simulink model "NonLinear_Plant"  (R2018a)
settings: Solver=VariableStepAuto  StartTime=0.0  StopTime=10.0  RelTol=1e-3
values from neighbouring files (symbols this model uses):
  Beta = 2.29e-06    [Plantvw.m]
  d = d    [Plantvw.m]
  dw = dw    [Plantsdv.m]    (also in Plantvw.m; Plantww.m)
  Kb = Kt    (= 0.0046)    [Plantvw.m]
  Kg = 50    [Plantvw.m]
  Kt = 0.0046    [Plantvw.m]
  La = 1.729e-03    (= 0.001729)    [Plantvw.m]
  mc = 2.76 + md    [Plantvw.m]
  R = R    [Plantww.m]
  Ra = 5.51    [Plantvw.m]
undefined symbols (not defined in the file or in its folder): Ad, Bd
settings Model: Creator=shravan  LastModifiedBy=shravan

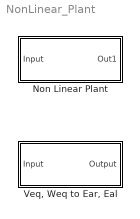
== system NonLinear_Plant ==
  "Non Linear Plant " : Subsystem
  "Veq, Weq to Ear, Eal " : Subsystem

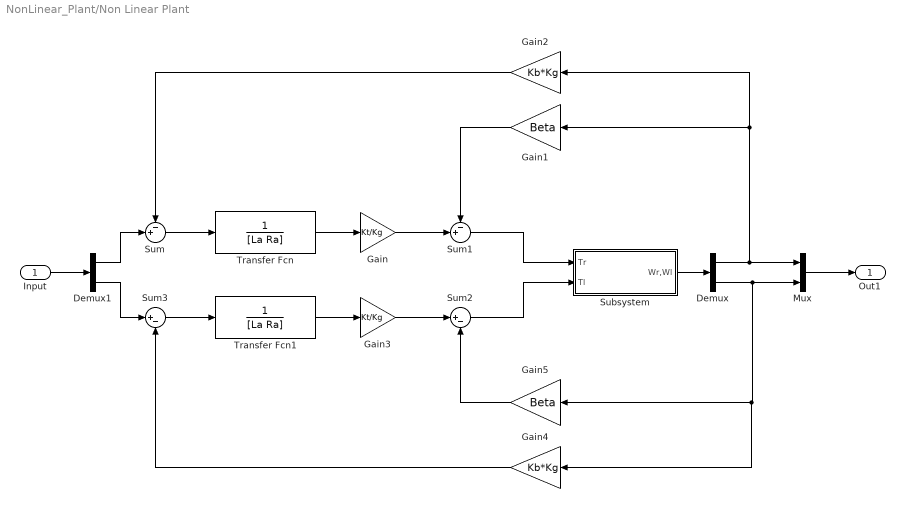
== system NonLinear_Plant/Non Linear Plant  ==
  Input : Inport
  Demux : Demux  Outputs=2
  Demux1 : Demux  Outputs=2
  Gain : Gain  Gain=Kt/Kg
  Gain1 : Gain  Gain=Beta
  Gain2 : Gain  Gain=Kb*Kg
  Gain3 : Gain  Gain=Kt/Kg
  Gain4 : Gain  Gain=Kb*Kg
  Gain5 : Gain  Gain=Beta
  Mux : Mux  Inputs=2
  Subsystem : Subsystem
  Sum : Sum  Inputs=-+|
  Sum1 : Sum  Inputs=-+|
  Sum2 : Sum  Inputs=|+-
  Sum3 : Sum  Inputs=|+-
  Transfer Fcn : TransferFcn  Denominator=[La Ra]
  Transfer Fcn1 : TransferFcn  Denominator=[La Ra]
  Out1 : Outport
  wires:
  Gain5/1 -> Sum2/2
  Gain4/1 -> Sum3/2
  Sum/1 -> Transfer Fcn/1
  Demux1/2 -> Sum3/1
  Gain1/1 -> Sum1/1
  Demux/1 -> Mux/1, Gain2/1, Gain1/1
  Subsystem/1(Wr,Wl) -> Demux/1
  Demux1/1 -> Sum/2
  Sum3/1 -> Transfer Fcn1/1
  Mux/1 -> Out1/1
  Gain2/1 -> Sum/1
  Gain/1 -> Sum1/2
  Input/1 -> Demux1/1
  Sum1/1 -> Subsystem/1(Tr)
  Transfer Fcn/1 -> Gain/1
  Transfer Fcn1/1 -> Gain3/1
  Gain3/1 -> Sum2/1
  Demux/2 -> Mux/2, Gain4/1, Gain5/1
  Sum2/1 -> Subsystem/2(Tl)

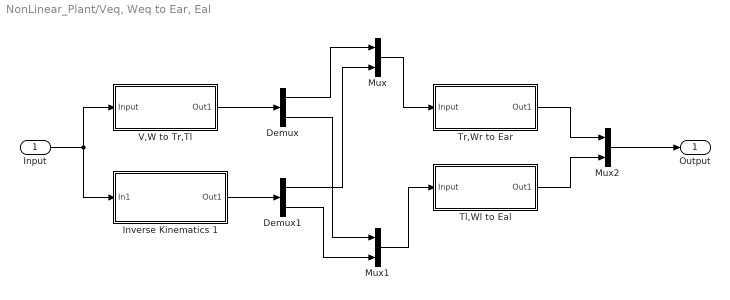
== system NonLinear_Plant/Veq, Weq to Ear, Eal  ==
  Input : Inport
  Demux : Demux  Outputs=2
  Demux1 : Demux  Outputs=2
  Inverse Kinematics 1 : Subsystem
  Mux : Mux  Inputs=2
  Mux1 : Mux  Inputs=2
  Mux2 : Mux  Inputs=2
  Tl,Wl to Eal : Subsystem
  Tr,Wr to Ear : Subsystem
  V,W to Tr,Tl : Subsystem
  Output : Outport
  wires:
  V,W to Tr,Tl/1(Out1) -> Demux/1
  Demux/1 -> Mux/1
  Mux/1 -> Tr,Wr to Ear/1(Input)
  Input/1 -> Inverse Kinematics 1/1(In1), V,W to Tr,Tl/1(Input)
  Inverse Kinematics 1/1(Out1) -> Demux1/1
  Demux1/1 -> Mux/2
  Demux/2 -> Mux1/1
  Demux1/2 -> Mux1/2
  Mux1/1 -> Tl,Wl to Eal/1(Input)
  Tr,Wr to Ear/1(Out1) -> Mux2/1
  Tl,Wl to Eal/1(Out1) -> Mux2/2
  Mux2/1 -> Output/1

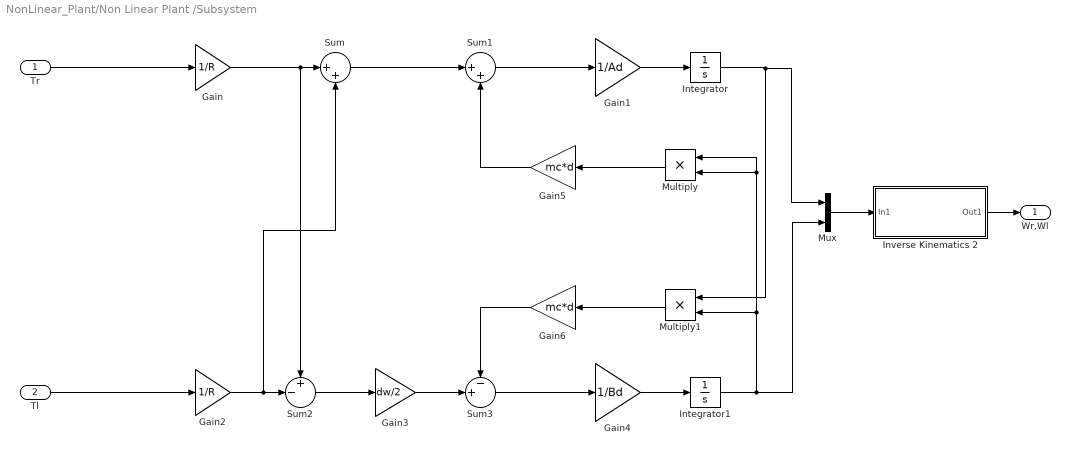
== system NonLinear_Plant/Non Linear Plant /Subsystem ==
  Tr : Inport
  Tl : Inport  Port=2
  Gain : Gain  Gain=1/R
  Gain1 : Gain  Gain=1/Ad
  Gain2 : Gain  Gain=1/R
  Gain3 : Gain  Gain=dw/2
  Gain4 : Gain  Gain=1/Bd
  Gain5 : Gain  Gain=mc*d
  Gain6 : Gain  Gain=mc*d
  Integrator : Integrator
  Integrator1 : Integrator
  Inverse Kinematics 2 : Subsystem
  Multiply : Product
  Multiply1 : Product
  Mux : Mux  Inputs=2
  Sum : Sum  Inputs=|++
  Sum1 : Sum  Inputs=|++
  Sum2 : Sum  Inputs=+-|
  Sum3 : Sum  Inputs=-+|
  Wr,Wl : Outport
  wires:
  Sum1/1 -> Gain1/1
  Multiply1/1 -> Gain6/1
  Sum3/1 -> Gain4/1
  Gain/1 -> Sum/1, Sum2/1
  Integrator/1 -> Mux/1, Multiply1/1
  Mux/1 -> Inverse Kinematics 2/1(In1)
  Gain4/1 -> Integrator1/1
  Inverse Kinematics 2/1(Out1) -> Wr,Wl/1
  Sum/1 -> Sum1/1
  Gain5/1 -> Sum1/2
  Tr/1 -> Gain/1
  Integrator1/1 -> Multiply1/2, Multiply/2, Multiply/1, Mux/2
  Multiply/1 -> Gain5/1
  Gain3/1 -> Sum3/2
  Sum2/1 -> Gain3/1
  Gain2/1 -> Sum/2, Sum2/2
  Gain6/1 -> Sum3/1
  Tl/1 -> Gain2/1
  Gain1/1 -> Integrator/1

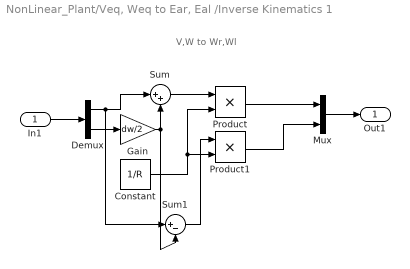
== system NonLinear_Plant/Veq, Weq to Ear, Eal /Inverse Kinematics 1 ==
  note: V,W to Wr,Wl
  In1 : Inport
  Constant : Constant  Value=1/R
  Demux : Demux  Outputs=2
  Gain : Gain  Gain=dw/2
  Mux : Mux  Inputs=2
  Product : Product
  Product1 : Product
  Sum : Sum  Inputs=|++
  Sum1 : Sum  Inputs=|+-
  Out1 : Outport
  wires:
  Mux/1 -> Out1/1
  In1/1 -> Demux/1
  Demux/2 -> Gain/1
  Demux/1 -> Sum1/1, Sum/1
  Sum/1 -> Product/1
  Constant/1 -> Product1/2, Product/2
  Sum1/1 -> Product1/1
  Product/1 -> Mux/1
  Product1/1 -> Mux/2
  Gain/1 -> Sum1/2, Sum/2

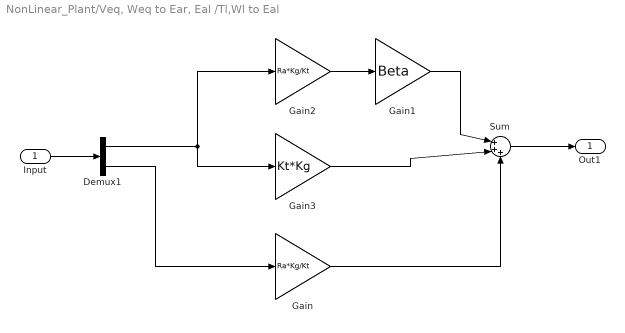
== system NonLinear_Plant/Veq, Weq to Ear, Eal /Tl,Wl to Eal ==
  Input : Inport
  Demux1 : Demux  Outputs=2
  Gain : Gain  Gain=Ra*Kg/Kt
  Gain1 : Gain  Gain=Beta
  Gain2 : Gain  Gain=Ra*Kg/Kt
  Gain3 : Gain  Gain=Kt*Kg
  Sum : Sum  Inputs=|+++
  Out1 : Outport
  wires:
  Demux1/1 -> Gain2/1, Gain3/1
  Gain/1 -> Sum/3
  Gain1/1 -> Sum/1
  Gain2/1 -> Gain1/1
  Input/1 -> Demux1/1
  Sum/1 -> Out1/1
  Demux1/2 -> Gain/1
  Gain3/1 -> Sum/2

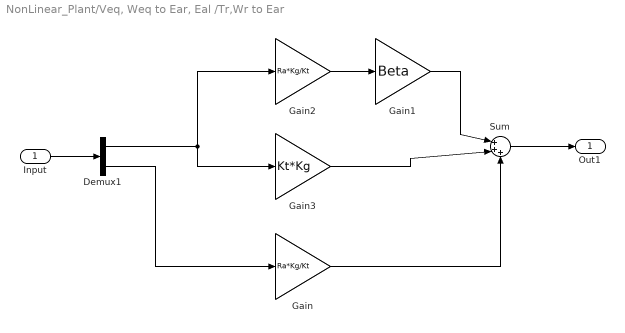
== system NonLinear_Plant/Veq, Weq to Ear, Eal /Tr,Wr to Ear ==
  Input : Inport
  Demux1 : Demux  Outputs=2
  Gain : Gain  Gain=Ra*Kg/Kt
  Gain1 : Gain  Gain=Beta
  Gain2 : Gain  Gain=Ra*Kg/Kt
  Gain3 : Gain  Gain=Kt*Kg
  Sum : Sum  Inputs=|+++
  Out1 : Outport
  wires:
  Demux1/1 -> Gain2/1, Gain3/1
  Gain/1 -> Sum/3
  Gain1/1 -> Sum/1
  Gain2/1 -> Gain1/1
  Input/1 -> Demux1/1
  Sum/1 -> Out1/1
  Demux1/2 -> Gain/1
  Gain3/1 -> Sum/2

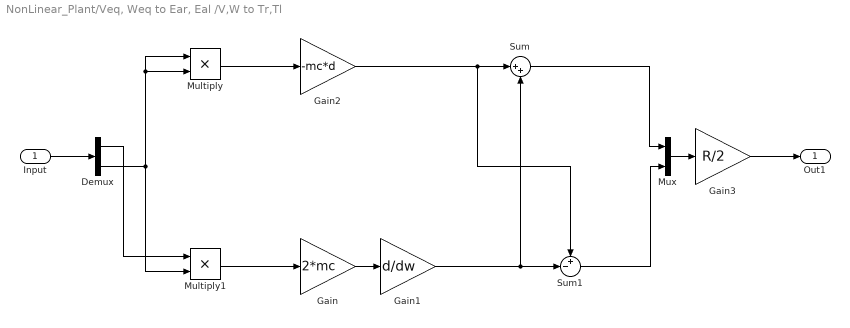
== system NonLinear_Plant/Veq, Weq to Ear, Eal /V,W to Tr,Tl ==
  Input : Inport
  Demux : Demux  Outputs=2
  Gain : Gain  Gain=2*mc
  Gain1 : Gain  Gain=d/dw
  Gain2 : Gain  Gain=-mc*d
  Gain3 : Gain  Gain=R/2
  Multiply : Product
  Multiply1 : Product
  Mux : Mux  Inputs=2
  Sum : Sum  Inputs=|++
  Sum1 : Sum  Inputs=+-|
  Out1 : Outport
  wires:
  Demux/1 -> Multiply1/1
  Mux/1 -> Gain3/1
  Gain/1 -> Gain1/1
  Input/1 -> Demux/1
  Multiply1/1 -> Gain/1
  Sum1/1 -> Mux/2
  Gain1/1 -> Sum1/2, Sum/2
  Gain2/1 -> Sum1/1, Sum/1
  Demux/2 -> Multiply1/2, Multiply/2, Multiply/1
  Gain3/1 -> Out1/1
  Multiply/1 -> Gain2/1
  Sum/1 -> Mux/1

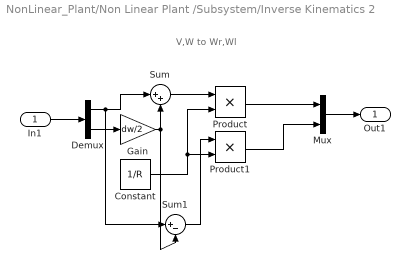
== system NonLinear_Plant/Non Linear Plant /Subsystem/Inverse Kinematics 2 ==
  note: V,W to Wr,Wl
  In1 : Inport
  Constant : Constant  Value=1/R
  Demux : Demux  Outputs=2
  Gain : Gain  Gain=dw/2
  Mux : Mux  Inputs=2
  Product : Product
  Product1 : Product
  Sum : Sum  Inputs=|++
  Sum1 : Sum  Inputs=|+-
  Out1 : Outport
  wires:
  Mux/1 -> Out1/1
  In1/1 -> Demux/1
  Demux/2 -> Gain/1
  Demux/1 -> Sum1/1, Sum/1
  Gain/1 -> Sum1/2, Sum/2
  Sum/1 -> Product/1
  Constant/1 -> Product1/2, Product/2
  Sum1/1 -> Product1/1
  Product/1 -> Mux/1
  Product1/1 -> Mux/2
